simulink model "Ilian_Buck"  (R2018a)
settings: Solver=ode23tb  StartTime=0.0  StopTime=0.2  MaxStep=10e-6  RelTol=1e-3
libraries: powerlib x12, powerlib_meascontrol x1
settings Model: Creator=Ilian  LastModifiedBy=ivank
settings SolverCC: InitialStep=10e-8

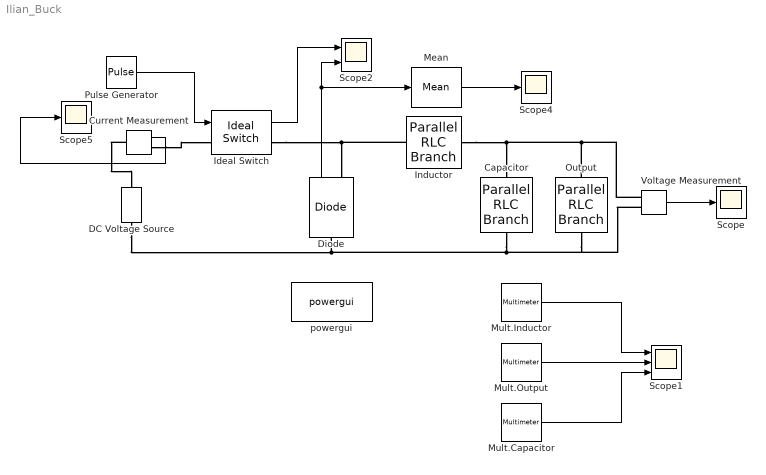
== system Ilian_Buck ==
  Capacitor : powerlib/Elements/Parallel RLC Branch  LConnTagsString=a  RConnTagsString=__new0  BranchType=C  Resistance=0  Inductance=1e-3  SetiL0=off  InitialCurrent=0  Capacitance=2.46e-6  Setx0=off  InitialVoltage=0  Measurements=Branch voltage and current
  Current Measurement : powerlib/Measurements/Current Measurement  PhasorSimulation=off  OutputType=Complex  PSBequivalent=0
  DC Voltage Source : powerlib/Electrical Sources/DC Voltage Source  Amplitude=200  Measurements=None
  Diode : powerlib/Power Electronics/Diode  Ron=0.001  Lon=0  Vf=0.8  IC=0  UseSnubber=0  Rs=500  Cs=250e-9  Measurements=on
  Ideal Switch : powerlib/Power Electronics/Ideal Switch  Ron=0.001  Lon=0  IC=0  Rs=1e5  Cs=inf  Measurements=on
  Inductor : powerlib/Elements/Parallel RLC Branch  LConnTagsString=a  RConnTagsString=__new0  BranchType=L  Resistance=0  Inductance=22e-3  SetiL0=off  InitialCurrent=0  Capacitance=0  Setx0=off  InitialVoltage=0  Measurements=Branch voltage and current
  Mean : powerlib_meascontrol/Measurements/Mean  Freq=5000  Vinit=0  Ts=0
  Mult.Capacitor : powerlib/Measurements/Multimeter  PhasorSimulation=off  OutputType=Complex  sel=[1 4]  L=6  Gain=[1 1]  yselected={'Ub: Capacitor','Ib: Capacitor'};  PSBOutputType=1  PSBequivalent=0  AxesSetting=[0,0.1,-100,100]  Display=0  SavedBlockNames=-11
  Mult.Inductor : powerlib/Measurements/Multimeter  PhasorSimulation=off  OutputType=Complex  sel=[2 5 1 4 3 6]  L=6  Gain=[1 1 1 1 1 1]  yselected={'Ub: Inductor','Ib: Inductor','Ub: Capacitor','Ib: Capacitor','Ub: Output','Ib: Output'};  PSBOutputType=1  PSBequivalent=0  AxesSetting=[0,0.1,-100,100]  Display=1  SavedBlockNames=-11
  Mult.Output : powerlib/Measurements/Multimeter  PhasorSimulation=off  OutputType=Complex  sel=[3 6]  L=6  Gain=[1 1]  yselected={'Ub: Output','Ib: Output'};  PSBOutputType=1  PSBequivalent=0  AxesSetting=[0,0.1,-100,100]  Display=0  SavedBlockNames=-11
  Output : powerlib/Elements/Parallel RLC Branch  LConnTagsString=a  RConnTagsString=__new0  BranchType=R  Resistance=7.225/3  Inductance=200e-3  SetiL0=off  InitialCurrent=0  Capacitance=100*10e-6  Setx0=off  InitialVoltage=0  Measurements=Branch voltage and current
  Pulse Generator : DiscretePulseGenerator  PulseType=Time based  Amplitude=5  Period=1/(581*10)  PulseWidth=85
  Scope : Scope
  Scope1 : Scope  NumInputPorts=3
  Scope2 : Scope  NumInputPorts=2
  Scope4 : Scope
  Scope5 : Scope
  Voltage Measurement : powerlib/Measurements/Voltage Measurement  PhasorSimulation=off  OutputType=Complex  PSBequivalent=0
  powergui : powerlib/powergui  Priority=1  SimulationMode=Continuous  SampleTime=50e-6  frequency=60  Iterations=50  frequencyindice=0  Pbase=100e6  ErrMax=1e-4  UnitsV=kV  UnitsW=MW  buscounter=0  FunctionMessages=off  echomessages=off  EnableUseOfTLC=off  CurrentSourceSwitches=off  DisableSnubberDevices=off  DisableRonSwitches=off  DisableVfSwitches=off  DisplayEquations=off  SolverType=Tustin/Backward Euler (TBE)  Interpol=off  ExternalGateDelay=off  methode=off  Ts=100  x0status=blocks  SPID=on  SwTol=0  HookPort=off  RestoreLinks=warning  ResistiveCurrentMeasurement=off  Frange=[0:2:500]  Ylog=off  Xlog=on  ShowGrid=off  save=off  variable=ZData  structure=0  ZoomFFT=off  StartTime=0.0  cycles=1  DisplayStyle=1  fundamental=60  FreqAxis=off  MaxFrequency=1000  frequencyindicesteady=1  RmsSteady=1  display=off
  wires:
  Voltage Measurement/1 -> Scope/1
  Mult.Inductor/1 -> Scope1/1
  Mult.Output/1 -> Scope1/2
  Mult.Capacitor/1 -> Scope1/3
  Diode/1 -> Mean/1, Scope2/2
  Pulse Generator/1 -> Ideal Switch/1
  Ideal Switch/1 -> Scope2/1
  Mean/1 -> Scope4/1
  Current Measurement/1 -> Scope5/1
  connections:
  Inductor/LConn1 -- Ideal Switch/RConn1 -- Diode/RConn1
  DC Voltage Source/LConn1 -- Output/RConn1 -- Voltage Measurement/LConn2 -- Capacitor/RConn1 -- Diode/LConn1
  Output/LConn1 -- Inductor/RConn1 -- Capacitor/LConn1 -- Voltage Measurement/LConn1
  Current Measurement/LConn1 -- DC Voltage Source/RConn1
  Current Measurement/RConn1 -- Ideal Switch/LConn1
